simulink model "boost"  (R2020b)
settings: Solver=VariableStepAuto  StartTime=0.0  StopTime=0.25  MaxStep=1e-6  RelTol=1e-3
libraries: powerlib x12
settings Model: Creator=shashank Pathak  LastModifiedBy=shashank Pathak

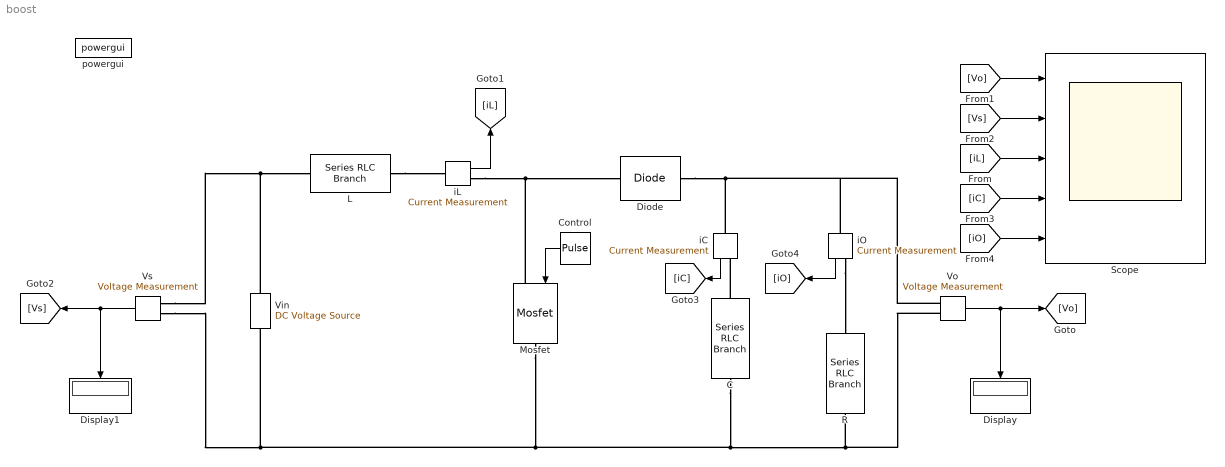
== system boost ==
  C : powerlib/Elements/Series RLC Branch  LConnTagsString=__new0  RConnTagsString=__new0  BranchType=C  Resistance=1  Inductance=1e-3  SetiL0=off  InitialCurrent=0  Capacitance=3e-5  Setx0=off  InitialVoltage=0  Measurements=None
  Control : DiscretePulseGenerator  PulseType=Time based  Period=1/25000  PulseWidth=75
  Diode : powerlib/Power Electronics/Diode  Ron=0  Lon=0  Vf=0  IC=0  UseSnubber=0  Rs=500  Cs=250e-9  Measurements=off
  Display : Display
  Display1 : Display
  L : powerlib/Elements/Series RLC Branch  LConnTagsString=__new0  RConnTagsString=__new0  BranchType=L  Resistance=1  Inductance=1.875e-4  SetiL0=off  InitialCurrent=0  Capacitance=1e-6  Setx0=off  InitialVoltage=0  Measurements=None
  Mosfet : powerlib/Power Electronics/Mosfet  Ron=0  Lon=0  Rd=0  Vfd=0  IC=0  Rs=1e5  Cs=inf  Measurements=off
  R : powerlib/Elements/Series RLC Branch  LConnTagsString=__new0  RConnTagsString=__new0  BranchType=R  Resistance=10  Inductance=1e-3  SetiL0=off  InitialCurrent=0  Capacitance=1e-6  Setx0=off  InitialVoltage=0  Measurements=None
  Scope : Scope  NumInputPorts=5
  Vin : powerlib/Electrical Sources/DC Voltage Source  Amplitude=5  Measurements=None
  Vo : powerlib/Measurements/Voltage Measurement  PhasorSimulation=off  OutputType=Complex  PSBequivalent=0
  Vs : powerlib/Measurements/Voltage Measurement  PhasorSimulation=off  OutputType=Complex  PSBequivalent=0
  iC : powerlib/Measurements/Current Measurement  PhasorSimulation=off  OutputType=Complex  PSBequivalent=0
  iL : powerlib/Measurements/Current Measurement  PhasorSimulation=off  OutputType=Complex  PSBequivalent=0
  iO : powerlib/Measurements/Current Measurement  PhasorSimulation=off  OutputType=Complex  PSBequivalent=0
  powergui : powerlib/powergui  Priority=1  SimulationMode=Continuous  SampleTime=50e-6  frequency=60  Iterations=50  frequencyindice=0  Pbase=100e6  ErrMax=1e-4  UnitsV=kV  UnitsW=MW  buscounter=0  FunctionMessages=off  echomessages=off  EnableUseOfTLC=off  CurrentSourceSwitches=off  DisableSnubberDevices=off  DisableRonSwitches=off  DisableVfSwitches=off  DisplayEquations=off  AutomaticDiscreteSolvers=off  SolverType=Tustin/Backward Euler (TBE)  Interpol=off  ExternalGateDelay=off  methode=off  Ts=100  x0status=blocks  SPID=on  SwTol=0  HookPort=off  NonlinearTolerance=1e-4  nMaxIteration=100  ContinueOnMaxIteration=off  RestoreLinks=warning  ResistiveCurrentMeasurement=off  Frange=[0:2:500]  Ylog=off  Xlog=on  ShowGrid=off  save=off  variable=ZData  structure=0  ZoomFFT=off  StartTime=0.0  cycles=1  DisplayStyle=1  fundamental=60  FreqAxis=off  MaxFrequency=1000  frequencyindicesteady=1  RmsSteady=1  display=off
  wires:
  [Vo] -> Scope/1
  [Vs] -> Scope/2
  [iL] -> Scope/3
  Vo/1 -> [Vo], Display/1
  iL/1 -> [iL]
  Vs/1 -> [Vs], Display1/1
  Control/1 -> Mosfet/1
  [iC] -> Scope/4
  iC/1 -> [iC]
  [iO] -> Scope/5
  iO/1 -> [iO]
  connections:
  Vin/RConn1 -- Vs/LConn1 -- L/LConn1
  iL/RConn1 -- Diode/LConn1 -- Mosfet/LConn1
  Diode/RConn1 -- iO/LConn1 -- Vo/LConn1 -- iC/LConn1
  C/RConn1 -- Vo/LConn2 -- R/RConn1 -- Mosfet/RConn1 -- Vin/LConn1 -- Vs/LConn2
  L/RConn1 -- iL/LConn1
  C/LConn1 -- iC/RConn1
  iO/RConn1 -- R/LConn1
